simulink model "playback_data"  (R2015a)
settings: Solver=FixedStepDiscrete  SolverMode=SingleTasking  StartTime=76  StopTime=110  FixedStep=sample_time  RelTol=1e-3
undefined symbols (not defined in the file): A1_notch_f1, A2_notch_f1, A_kalman_swing_load, A_kalman_transverse, A_kalman_vertical, A_lpf_accelerometer, A_lpf_dtau, A_lpf_fourbar_angles, A_lpf_imu, A_lpf_lateral_angle, B1_lpf_accelerometer, B1_lpf_dtau, B1_lpf_fourbar_angles, B1_lpf_imu, B1_lpf_lateral_angle, B1_notch_f1, B2_lpf_accelerometer, B2_lpf_dtau, B2_lpf_fourbar_angles, B2_lpf_imu, B2_lpf_lateral_angle, B2_notch_f1, B_dx_versus_x0, B_kalman_swing_load, B_kalman_transverse, B_kalman_vertical, backwards_K_sag_of_t, backwards_P_sag_of_t, C_kalman_swing_load, C_kalman_transverse, C_kalman_vertical, com_leg_motor, com_torso, contact_threshold, control_start_time, d_ankle_to_foot, d_vertical_com, desired_com_forward_velocity, desired_com_lateral_velocity, desired_initial_leg_roll_left, desired_initial_leg_roll_right, desired_stance_beta2, desired_standing_torso_pitch, desired_standing_torso_roll, desired_standing_z, desired_torso_pitch, desired_torso_roll, Discrete, enable_bouncing, fcut_contact, fdesignblkfcn, forward_dx_of_dxstar, forward_x_of_dxstar, g, gcbh, HIP_MTR_MAX_CONT_TORQUE, HIP_MTR_MAX_TORQUE, i_leg_motor, i_robot, i_torso ... (+78)
libraries: simulink x65, dsparch4 x18, ctrlSharedLib x14, dspfdesign x4
(part 13 of 13)

== matlab function playback_data/Control1/Behavior Control/Compute COM Translational Acceleration (IMU uses non-rotating measurement frame) ==
  data: com_acceleration_world output; torso_angular_accelerations input; imu_translational_accelerations_body input; torso_roll input; torso_pitch input; torso_yaw input; com_position_world input; com_velocity_world input; hip_roll_accelerations input; right_hip_roll input; left_hip_roll input; pelvis_to_imu parameter; com_torso parameter; com_leg_motor parameter; m_leg_motor parameter; m_leg parameter; m_torso parameter; torso_com_acceleration_world output; pelvis_acceleration_world output; right_hip_acceleration_world output; left_hip_acceleration_world output; com_acceleration_yawed output; g parameter
function [com_acceleration_world, torso_com_acceleration_world, pelvis_acceleration_world, right_hip_acceleration_world, left_hip_acceleration_world, com_acceleration_yawed] ...
          = compute_com_acceleration(torso_angular_accelerations, imu_translational_accelerations_body, torso_roll, torso_pitch, torso_yaw, ...
          com_position_world, com_velocity_world, ...
          hip_roll_accelerations, right_hip_roll, left_hip_roll, pelvis_to_imu, com_torso, com_leg_motor, m_leg_motor, m_leg, m_torso, g)

    % Body frame to Yawed frame rotations  
    R_body_to_yawed = R_pitch(torso_pitch(1))*R_roll(torso_roll(1));
    dR_body_to_yawed = dR_pitch(torso_pitch(1),torso_pitch(2))*R_roll(torso_roll(1)) + R_pitch(torso_pitch(1))*dR_roll(torso_roll(1),torso_roll(2));
    ddR_body_to_yawed = ddR_pitch(torso_pitch(1),torso_pitch(2),torso_angular_accelerations(2))*R_roll(torso_roll(1)) ...
                        + R_pitch(torso_pitch(1))*ddR_roll(torso_roll(1),torso_roll(2),torso_angular_accelerations(1)) ... 
                        + 2*dR_pitch(torso_pitch(1),torso_pitch(2))*dR_roll(torso_roll(1),torso_roll(2));
    % Yawed frame to World frame rotations  
    R_yawed_to_world = R_yaw(torso_yaw(1));
    dR_yawed_to_world = dR_yaw(torso_yaw(1),torso_yaw(2));
    ddR_yawed_to_world = ddR_yaw(torso_yaw(1),torso_yaw(2),torso_angular_accelerations(3));
    % Compute translational acceleration of torso COM
    R_position_body_to_world = R_yawed_to_world*R_body_to_yawed;
    R_velocity_body_to_world = dR_yawed_to_world*R_body_to_yawed + R_yawed_to_world*dR_body_to_yawed;
    R_acceleration_body_to_world = ddR_yawed_to_world*R_body_to_yawed + 2*dR_yawed_to_world*dR_body_to_yawed + R_yawed_to_world*ddR_body_to_yawed;
    imu_to_torso_com_acceleration_world = R_acceleration_body_to_world*(com_torso - pelvis_to_imu)';
    imu_acceleration_world = R_yawed_to_world*R_body_to_yawed*imu_translational_accelerations_body;
    torso_com_acceleration_world = imu_acceleration_world + imu_to_torso_com_acceleration_world;
    % Compute accelerations of hip COMs
    R_right_hip_to_body =     R_roll(-pi/2+right_hip_roll(1));
    dR_right_hip_to_body =   dR_roll(-pi/2+right_hip_roll(1), right_hip_roll(2));
    ddR_right_hip_to_body = ddR_roll(-pi/2+right_hip_roll(1), right_hip_roll(2), hip_roll_accelerations(1));
    R_left_hip_to_body =     R_roll(pi/2-left_hip_roll(1));
    dR_left_hip_to_body =   dR_roll(pi/2-left_hip_roll(1), -left_hip_roll(2));
    ddR_left_hip_to_body = ddR_roll(pi/2-left_hip_roll(1), -left_hip_roll(2), -hip_roll_accelerations(2));
    imu_to_pelvis_com_acceleration_world = R_acceleration_body_to_world*(-pelvis_to_imu)';  
    pelvis_acceleration_world = imu_acceleration_world + imu_to_pelvis_com_acceleration_world;
    left_hip_acceleration_world = pelvis_acceleration_world + (R_acceleration_body_to_world*R_left_hip_to_body + 2*R_velocity_body_to_world*dR_left_hip_to_body + R_position_body_to_world*ddR_left_hip_to_body)*com_leg_motor';
    right_hip_acceleration_world = pelvis_acceleration_world + (R_acceleration_body_to_world*R_right_hip_to_body + 2*R_velocity_body_to_world*dR_right_hip_to_body + R_position_body_to_world*ddR_right_hip_to_body)*(com_leg_motor.*[1,-1,1])';
    % Compute total system COM acceleration
    m_hip = m_leg+m_leg_motor;
    m_total = 2*m_hip + m_torso;
    com_acceleration_world = (m_torso*torso_com_acceleration_world + m_hip*(left_hip_acceleration_world + right_hip_acceleration_world))/m_total;
    com_acceleration_yawed = ddR_yawed_to_world'*com_position_world + 2*dR_yawed_to_world'*com_velocity_world + R_yawed_to_world'*com_acceleration_world;
    com_acceleration_yawed(3) = com_acceleration_yawed(3) - g;
end

function R_yp = R_pitch(theta) % map from pitched to yawed
  R_yp = [cos(theta), 0, sin(theta); ...
          0, 1, 0; ...
          -sin(theta), 0, cos(theta)];
end
function dR_yp = dR_pitch(theta,dtheta)
  dR_yp = dtheta*[-sin(theta), 0, cos(theta); ...
                  0, 0, 0; ... 
                  -cos(theta), 0, -sin(theta)];
end
function ddR_yp = ddR_pitch(theta,dtheta,ddtheta)
  ddR_yp = ddtheta*[-sin(theta), 0, cos(theta); ...
                    0, 0, 0; ... 
                    -cos(theta), 0, -sin(theta)] ...
           + dtheta^2*[-cos(theta), 0, -sin(theta); ...
                     0, 0, 0; ...
                     sin(theta), 0, -cos(theta)];
end
function R_pr = R_roll(phi) % map from rolled to pitched
  R_pr = [1, 0, 0; ...
          0, cos(phi), -sin(phi); ...
          0, sin(phi), cos(phi)]; 
end
function dR_pr = dR_roll(phi,dphi)
  dR_pr = dphi*[0, 0, 0; ...
                0, -sin(phi), -cos(phi); ...
                0, cos(phi), -sin(phi)];
end
function ddR_pr = ddR_roll(phi, dphi, ddphi)
  ddR_pr = ddphi*[0, 0, 0; ...
                  0, -sin(phi), -cos(phi); ...
                  0, cos(phi), -sin(phi)] ...
           + dphi^2*[0, 0, 0; ...
                   0, -cos(phi), sin(phi);...
                   0, -sin(phi), -cos(phi)];
end
function R_gy = R_yaw(psi) % map yawed frame to global
  R_gy = [cos(psi), -sin(psi), 0; sin(psi), cos(psi), 0; 0 0 1]; 
end
function dR_gy = dR_yaw(psi,dpsi)
  dR_gy = dpsi*[-sin(psi), -cos(psi), 0; cos(psi), -sin(psi), 0; 0 0 0];
end
function ddR_gy = ddR_yaw(psi,dpsi,ddpsi)
  ddR_gy = ddpsi*[-sin(psi), -cos(psi), 0; cos(psi), -sin(psi), 0; 0 0 0] ...
           + dpsi^2*[-cos(psi), sin(psi), 0; -sin(psi), -cos(psi), 0; 0 0 0];
end

== matlab function playback_data/Control1/Behavior Control/State Estimation/ComputeKneePositions ==
  data: roll input; pitch input; yaw input; left_leg_sagittal_angle input; left_leg_lateral_angle input; left_leg_length input; right_leg_sagittal_angle input; right_leg_lateral_angle input; right_leg_length input; right_back_angle input; left_back_angle input; right_front_angle input; left_front_angle input; m_torso parameter; m_leg_motor parameter; m_leg parameter; com_torso parameter; com_leg_motor parameter; lateral_offset parameter; front_knee_to_right_foot output; back_knee_to_right_foot output; front_knee_to_left_foot output; back_knee_to_left_foot output
function [front_knee_to_right_foot, back_knee_to_right_foot,...
          front_knee_to_left_foot, back_knee_to_left_foot] = ...
         KneePositionsUsingKinematics(roll, pitch, yaw, ...
                                    left_leg_sagittal_angle, left_leg_lateral_angle, left_leg_length, ...
                                    right_leg_sagittal_angle, right_leg_lateral_angle, right_leg_length, ...
                                    right_back_angle, left_back_angle, right_front_angle, left_front_angle,...
                                    m_torso, m_leg_motor, m_leg, com_torso, com_leg_motor, lateral_offset)
                    
    q =  [roll(1), pitch(1), yaw(1), left_leg_sagittal_angle(1), left_leg_lateral_angle(1), left_leg_length(1), right_leg_sagittal_angle(1), right_leg_lateral_angle(1), right_leg_length(1)];
    dq = [roll(2), pitch(2), yaw(2), left_leg_sagittal_angle(2), left_leg_lateral_angle(2), left_leg_length(2), right_leg_sagittal_angle(2), right_leg_lateral_angle(2), right_leg_length(2)];                
    [ ~, ~, left_foot_to_com, ~, right_foot_to_com, ~ ] = ComCalculationFromRobot( q, dq, m_torso, m_leg_motor, m_leg, com_torso, com_leg_motor, lateral_offset );

    q =  [roll(1), pitch(1), yaw(1), left_front_angle(1), left_leg_lateral_angle(1), 0.5, right_front_angle(1), right_leg_lateral_angle(1), 0.5];
    dq = [roll(2), pitch(2), yaw(2), left_front_angle(2), left_leg_lateral_angle(2), 0, right_front_angle(2), right_leg_lateral_angle(2), 0];   
    [ ~, ~, left_front_knee_to_com, ~, right_front_knee_to_com, ~ ] = ComCalculationFromRobot( q, dq, m_torso, m_leg_motor, m_leg, com_torso, com_leg_motor, lateral_offset );
    
    q =  [roll(1), pitch(1), yaw(1), left_back_angle(1), left_leg_lateral_angle(1), 0.4, right_back_angle(1), right_leg_lateral_angle(1), 0.4];
    dq = [roll(2), pitch(2), yaw(2), left_back_angle(2), left_leg_lateral_angle(2), 0, right_back_angle(2), right_leg_lateral_angle(2), 0];   
    [ ~, ~, left_back_knee_to_com, ~, right_back_knee_to_com, ~ ] = ComCalculationFromRobot( q, dq, m_torso, m_leg_motor, m_leg, com_torso, com_leg_motor, lateral_offset );
   
    front_knee_to_left_foot = left_front_knee_to_com(4:6) - left_foot_to_com(4:6);
    front_knee_to_right_foot = right_front_knee_to_com(4:6) - right_foot_to_com(4:6);
    back_knee_to_left_foot = left_back_knee_to_com(4:6) - left_foot_to_com(4:6);
    back_knee_to_right_foot = right_back_knee_to_com(4:6) - right_foot_to_com(4:6);
end

== matlab function playback_data/Control1/Behavior Control/State Estimation/Kalman Filtering/Measurement Noise Covariance Matricies ==
  data: R_transverse output; vertical_GRF_L input; vertical_GRF_R input; R_kalman_foot_stance parameter; R_kalman_foot_slip parameter; R_kalman_accelerometer parameter; sample_time parameter; m_total_real parameter; g parameter; R_vertical output; kalman_stance_slip_threshold parameter
function [R_transverse, R_vertical] =...
         MeasurementNoiseCovariance(vertical_GRF_L, vertical_GRF_R, ...
           R_kalman_foot_stance, R_kalman_foot_slip, R_kalman_accelerometer, sample_time, m_total_real, g, kalman_stance_slip_threshold)

    % filter states: [dx_w]; [dy_w]; [dz_w];
    % measurements:  [dx_w-dfL + dfL_hat; dx_w-dfR + dfR_hat]; 

    ratio_L = max(0, min(vertical_GRF_L/(kalman_stance_slip_threshold*m_total_real*g),1)); % ratio is 0 if no load, 1 if at least equilibrium
    ratio_R = max(0, min(vertical_GRF_R/(kalman_stance_slip_threshold*m_total_real*g),1));
    R_transverse = diag([ratio_L*R_kalman_foot_stance + (1-ratio_L)*R_kalman_foot_slip, ...
                         ratio_R*R_kalman_foot_stance + (1-ratio_R)*R_kalman_foot_slip, ...
                         R_kalman_accelerometer])/sample_time;
    R_vertical = diag([ratio_L*R_kalman_foot_stance  + (1-ratio_L)*R_kalman_foot_slip,...
                       ratio_R*R_kalman_foot_stance  + (1-ratio_R)*R_kalman_foot_slip,...
                       R_kalman_accelerometer])/sample_time;
end

== matlab function playback_data/Control1/Behavior Control/State Estimation/Kalman Filtering/eigen values ==
  data: Z input; E output
function E = eigen(Z)
    E = real(eig(Z));
    E = sort(E);
end

== matlab function playback_data/Control1/Behavior Control/State Estimation/Kalman Filtering/eigen values1 ==
  data: Z input; E output
function E = eigen(Z)
    E = real(eig(Z));
    E = sort(E);
end

== matlab function playback_data/Control1/Behavior Control/State Estimation/Kalman Filtering/eigen values2 ==
  data: Z input; E output
function E = eigen(Z)
    E = real(eig(Z));
    E = sort(E);
end

== matlab function playback_data/Control1/Behavior Control/State Estimation/PositionUsingRobotGeometry ==
  data: com_left_foot output; dcom_left_foot output; com_right_foot output; dcom_right_foot output; right_left input; horizontal_com_position output; roll input; pitch input; yaw input; horizontal_com_velocity output; lateral_com_position output; lateral_com_velocity output; left_leg_sagittal_angle input; left_leg_lateral_angle input; left_leg_length input; right_leg_sagittal_angle input; right_leg_lateral_angle input; right_leg_length input; m_torso parameter; m_leg_motor parameter; m_leg parameter; com_torso parameter; com_leg_motor parameter; lateral_offset parameter; vertical_com_position output; vertical_com_velocity output; com_pelvis output; dcom_pelvis output
% Returns 2D COM relative to primary foot
function [com_left_foot, dcom_left_foot, com_right_foot, dcom_right_foot,...
          horizontal_com_position, horizontal_com_velocity, ...
          lateral_com_position, lateral_com_velocity, ...
          vertical_com_position, vertical_com_velocity, ...
          com_pelvis, dcom_pelvis] = ...
         ComPositionUsingRobotGeometry(right_left, ...
                                    roll, pitch, yaw, ...
                                    left_leg_sagittal_angle, left_leg_lateral_angle, left_leg_length, ...
                                    right_leg_sagittal_angle, right_leg_lateral_angle, right_leg_length, ...
                                    m_torso, m_leg_motor, m_leg, com_torso, com_leg_motor, lateral_offset)
                    
    q =  [roll(1), pitch(1), yaw(1), left_leg_sagittal_angle(1), left_leg_lateral_angle(1), left_leg_length(1), right_leg_sagittal_angle(1), right_leg_lateral_angle(1), right_leg_length(1)];
    dq = [roll(2), pitch(2), yaw(2), left_leg_sagittal_angle(2), left_leg_lateral_angle(2), left_leg_length(2), right_leg_sagittal_angle(2), right_leg_lateral_angle(2), right_leg_length(2)];
                    
    [ com_pelvis, dcom_pelvis, ...
      com_left_foot, dcom_left_foot, ...
      com_right_foot, dcom_right_foot ] = ...
    ComCalculationFromRobot( q, dq, m_torso, m_leg_motor, m_leg, com_torso, com_leg_motor, lateral_offset );

    if right_left
        com_position = com_right_foot(4:6);
        com_velocity = dcom_right_foot(4:6);
    else
        com_position = com_left_foot(4:6);
        com_velocity = dcom_left_foot(4:6);
    end


    horizontal_com_position = com_position(1);
    horizontal_com_velocity = com_velocity(1);
    lateral_com_position = com_position(2);
    lateral_com_velocity = com_velocity(2);
    vertical_com_position = com_position(3);
    vertical_com_velocity = com_velocity(3);

end
